simulink model "LQR"  (R2021b)
settings: Solver=VariableStepAuto  StartTime=0.0  StopTime=10.0  RelTol=1e-3
values from neighbouring files (symbols this model uses):
  A = [-0.0345, 0.847, -2.950, -9.698; -0.513, -3.249, 19.340, -1.479; 0.278, -1.586, -3.233, 0; 0, 0, 1, 0]    [Control_Part.m]    (also in Dynamics_part_I.m = [0.5-410*lmbd, 410; -0.45, -401.8*lmbd])
  B = [0.465; -3.050; -28.910; 0]    [Control_Part.m]
  C_angle = [0,0,0,1]    [Control_Part.m]
  K = [0.823, 8.84, 16.89]    [Control_Part.m]
  Nbar = -inv(C_angle*inv(A-B*K)*B)    [Control_Part.m]
settings Model: Creator=İbrahim  LastModifiedBy=İbrahim

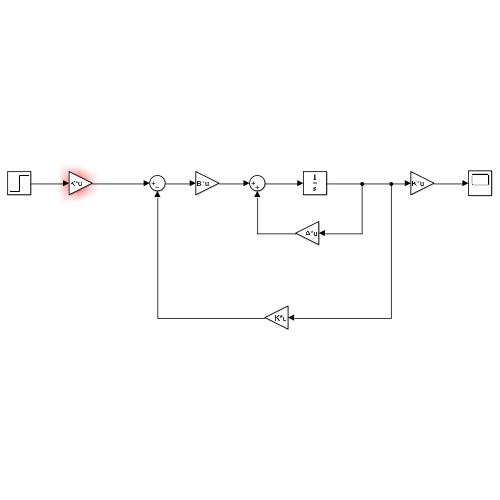
[thumbnail: Simulink's stored preview of the top-level diagram]
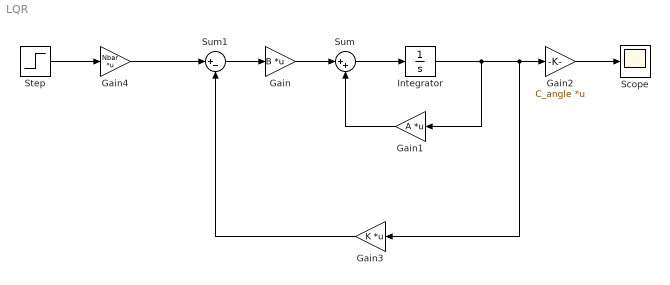
== system LQR ==
  Gain : Gain  Gain=B  Multiplication=Matrix(K*u)
  Gain1 : Gain  Gain=A  Multiplication=Matrix(K*u)
  Gain2 : Gain  Gain=C_angle  Multiplication=Matrix(K*u)
  Gain3 : Gain  Gain=K  Multiplication=Matrix(K*u)
  Gain4 : Gain  Gain=Nbar  Multiplication=Matrix(K*u)
  Integrator : Integrator
  Scope : Scope
  Step : Step  Time=0  After=0.1571  SampleTime=0
  Sum : Sum  Inputs=|++
  Sum1 : Sum  Inputs=|+-
  wires:
  Gain/1 -> Sum/1
  Gain1/1 -> Sum/2
  Sum/1 -> Integrator/1
  Integrator/1 -> Gain1/1, Gain3/1, Gain2/1
  Gain2/1 -> Scope/1
  Gain3/1 -> Sum1/2
  Sum1/1 -> Gain/1
  Gain4/1 -> Sum1/1
  Step/1 -> Gain4/1
